simulink model "LIF"  (R2024b)
settings: Solver=ode23t  StartTime=0.0  StopTime=3  MaxStep=1e-05
libraries: fl_lib x15, nesl_utility x5
settings Model: SimulationMode=accelerator  Creator=georg  LastModifiedBy=georg
settings SolverCC: SolverResetMethod=Robust  AutoInsertRateTranBlk=on

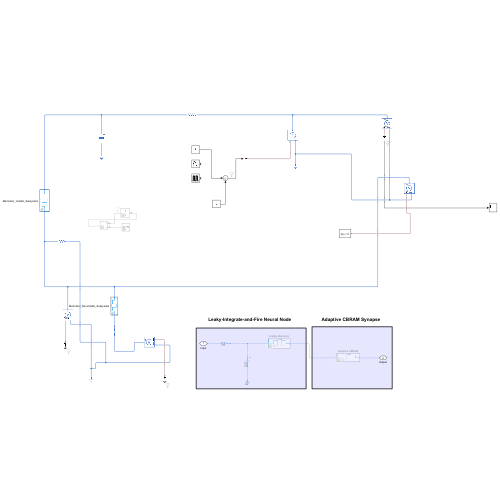
[thumbnail: Simulink's stored preview of the top-level diagram]
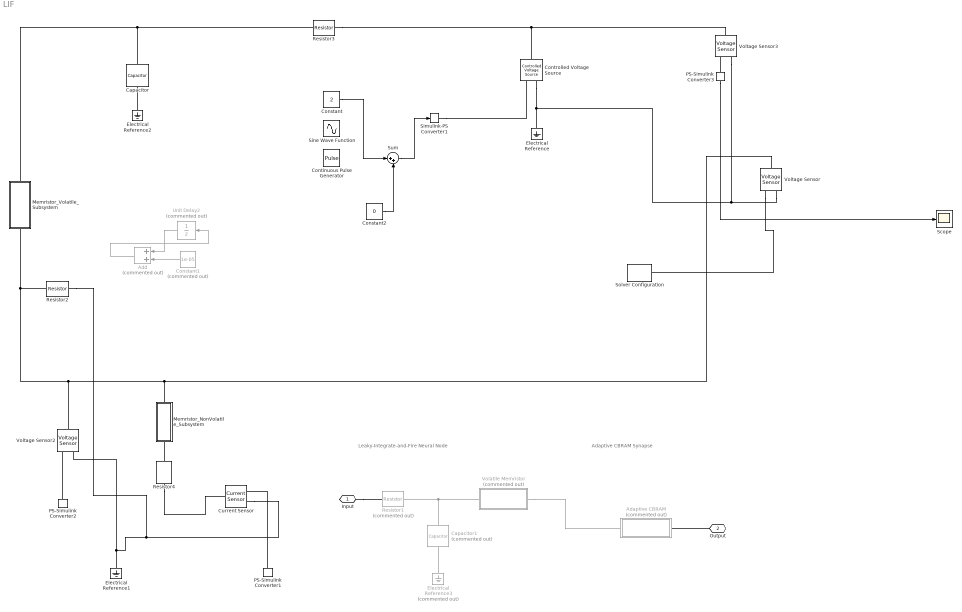
== system LIF ==
  note: Leaky-Integrate-and-Fire Neural Node
  note: Adaptive CBRAM Synapse
  Adaptive CBRAM : Subsystem  Commented=on  ReferencedSubsystem=Memristor_NonVolatile_Subsystem
  Add : Sum  Commented=on
  Capacitor : fl_lib/Electrical/Electrical Elements/Capacitor  c=150 nF  r=1e-6 Ohm  g=0 1/Ohm  i_specify=off  i_priority=None  i=0 A  i_nominal_specify=off  i_nominal_value=1  i_nominal_unit=A  v_specify=off  v_priority=None  v=0 V  v_nominal_specify=off  v_nominal_value=1  v_nominal_unit=V  vc_specify=off  vc_priority=High  vc=0 V  vc_nominal_specify=off  vc_nominal_value=1  vc_nominal_unit=V
  Capacitor1 : fl_lib/Electrical/Electrical Elements/Capacitor  Commented=on  c=150 nF  r=1e-6 Ohm  g=0 1/Ohm  i_specify=off  i_priority=None  i=0 A  i_nominal_specify=off  i_nominal_value=1  i_nominal_unit=A  v_specify=off  v_priority=None  v=0 V  v_nominal_specify=off  v_nominal_value=1  v_nominal_unit=V  vc_specify=off  vc_priority=High  vc=0 V  vc_nominal_specify=off  vc_nominal_value=1  vc_nominal_unit=V
  Constant : Constant  Value=2
  Constant1 : Constant  Commented=on  Value=1e-05
  Constant2 : Constant  Value=0
  Continuous Pulse Generator : DiscretePulseGenerator  PulseType=Time based  Amplitude=2  Period=0.1  PulseWidth=50
  Controlled Voltage Source : fl_lib/Electrical/Electrical Sources/Controlled Voltage Source
  Current Sensor : fl_lib/Electrical/Electrical Sensors/Current Sensor
  Electrical Reference : fl_lib/Electrical/Electrical Elements/Electrical Reference
  Electrical Reference1 : fl_lib/Electrical/Electrical Elements/Electrical Reference
  Electrical Reference2 : fl_lib/Electrical/Electrical Elements/Electrical Reference
  Electrical Reference3 : fl_lib/Electrical/Electrical Elements/Electrical Reference  Commented=on
  Memristor_NonVolatile_Subsystem : Subsystem  ReferencedSubsystem=Memristor_NonVolatile_Subsystem
  Memristor_Volatile_Subsystem : Subsystem  ReferencedSubsystem=Memristor_Volatile_Subsystem
  PS-Simulink Converter1 : nesl_utility/PS-Simulink Converter  PhysicalDomain=network_engine_domain  SubClassName=ps_output  LeftPortType=input  RightPortType=output  PseudoPeriodic=off  Frequencies=[]  VectorFormat=inherit  Unit=inherit  AffineConversion=off
  PS-Simulink Converter2 : nesl_utility/PS-Simulink Converter  PhysicalDomain=network_engine_domain  SubClassName=ps_output  LeftPortType=input  RightPortType=output  PseudoPeriodic=off  Frequencies=[]  VectorFormat=inherit  Unit=inherit  AffineConversion=off
  PS-Simulink Converter3 : nesl_utility/PS-Simulink Converter  PhysicalDomain=network_engine_domain  SubClassName=ps_output  LeftPortType=input  RightPortType=output  PseudoPeriodic=off  Frequencies=[]  VectorFormat=inherit  Unit=inherit  AffineConversion=off
  Resistor1 : fl_lib/Electrical/Electrical Elements/Resistor  Commented=on  R=475 kOhm  i_specify=off  i_priority=None  i=0 A  i_nominal_specify=off  i_nominal_value=1  i_nominal_unit=A  v_specify=off  v_priority=None  v=0 V  v_nominal_specify=off  v_nominal_value=1  v_nominal_unit=V
  Resistor2 : fl_lib/Electrical/Electrical Elements/Resistor  R=0.3 MOhm  i_specify=off  i_priority=None  i=0 A  i_nominal_specify=off  i_nominal_value=1  i_nominal_unit=A  v_specify=off  v_priority=None  v=0 V  v_nominal_specify=off  v_nominal_value=1  v_nominal_unit=V
  Resistor3 : fl_lib/Electrical/Electrical Elements/Resistor  R=475 kOhm  i_specify=off  i_priority=None  i=0 A  i_nominal_specify=off  i_nominal_value=1  i_nominal_unit=A  v_specify=off  v_priority=None  v=0 V  v_nominal_specify=off  v_nominal_value=1  v_nominal_unit=V
  Resistor4 : fl_lib/Electrical/Electrical Elements/Resistor  R=10 kOhm  i_specify=off  i_priority=None  i=0 A  i_nominal_specify=off  i_nominal_value=1  i_nominal_unit=A  v_specify=off  v_priority=None  v=0 V  v_nominal_specify=off  v_nominal_value=1  v_nominal_unit=V
  Scope : Scope
  Simulink-PS Converter1 : nesl_utility/Simulink-PS Converter  PhysicalDomain=network_engine_domain  SubClassName=ps_input  LeftPortType=input  RightPortType=output  PseudoPeriodic=off  Frequencies=[]  NoiseDistribution=none  NoiseParameters=[]  Unit=1  AffineConversion=off  FilteringAndDerivatives=filter  SimscapeFilterOrder=1  InputFilterTimeConstant=0.00001  UdotUserProvided=0
  Sine Wave Function : Sin  Amplitude=2  SampleTime=0
  Solver Configuration : nesl_utility/Solver Configuration  PhysicalDomain=network_engine_domain  SubClassName=solver  LeftPortType=input  RightPortType=generic  Tones=[]  Harmonics=[]  SimulateNoise=off  Profile=off  UseLocalSampling=off  EnableSwitchedLinearOptims=on  FrequencyDomain=off  UseCCode=off  RelTol=0.001  AbsTol=0.001  MinStep=1e-09  ToWorkspace=off  RevertToSquareIcSolve=off  NumHomotopyIterations=100  PhasorMode=off  PhasorModeNumHarmonics=1  ConsistencySolver=NEWTON_XTOL_AFTER_FTOL  IndexReductionMethod=DerivativeReplacement  DoDC=off  ResidualTolerance=1e-09  ConsistencyTolSource=GLOBAL  ConsistencyAbsTol=0.001  ConsistencyRelTol=0.001  ConsistencyTolFactor=0.001  UseLocalSolver=off  LocalSolverChoice=NE_BACKWARD_EULER_ADVANCER  ResolveIndetEquations=on  FunctionEvalNumThread=1  LocalSolverSampleTime=0.001  DoFixedCost=off  MaxNonlinIter=3  MaxModeIter=2  ComputeImpulses=off  ImpulseIterations=2  LinearAlgebra=auto  LinearAlgebraNumThread=0  EquationFormulation=NE_TIME_EF  DelaysMemoryBudget=1024  AutomaticFiltering=on  FilteringTimeConstant=0.001  PartitionStorageMethod=AS_NEEDED  PartitionMemoryBudget=1024  PartitionMethod=ROBUST  MultibodyUseLocalSolver=off  MultibodyLocalSolverChoice=ODE1  MultibodyLocalSolverSampleTime=0.001
  Sum : Sum  Inputs=|++
  Unit Delay2 : UnitDelay  Commented=on  SampleTime=1e-05  HasFrameUpgradeWarning=on
  Volatile Memristor : Subsystem  Commented=on  ReferencedSubsystem=Memristor_Volatile_Subsystem
  Voltage Sensor : fl_lib/Electrical/Electrical Sensors/Voltage Sensor
  Voltage Sensor2 : fl_lib/Electrical/Electrical Sensors/Voltage Sensor
  Voltage Sensor3 : fl_lib/Electrical/Electrical Sensors/Voltage Sensor
  Input : PMIOPort  Side=Left
  Output : PMIOPort  Port=2  Side=Left
  wires:
  PS-Simulink Converter3/1 -> Scope/1
  Constant1/1 -> Add/2
  Unit Delay2/1 -> Add/1
  Add/1 -> Unit Delay2/1
  Constant2/1 -> Sum/2
  Sum/1 -> Simulink-PS Converter1/1
  Constant/1 -> Sum/1
  connections:
  Voltage Sensor/RConn2 -- Voltage Sensor3/RConn2 -- Controlled Voltage Source/RConn2 -- Electrical Reference/LConn1
  Voltage Sensor/RConn1 -- Solver Configuration/RConn1
  Memristor_Volatile_Subsystem/LConn1 -- Capacitor/LConn1 -- Resistor3/LConn1
  Electrical Reference1/LConn1 -- Current Sensor/RConn2 -- Resistor2/RConn1 -- Voltage Sensor2/RConn2
  PS-Simulink Converter2/LConn1 -- Voltage Sensor2/RConn1
  Electrical Reference2/LConn1 -- Capacitor/RConn1
  Controlled Voltage Source/LConn1 -- Resistor3/RConn1 -- Voltage Sensor3/LConn1
  PS-Simulink Converter3/LConn1 -- Voltage Sensor3/RConn1
  Simulink-PS Converter1/RConn1 -- Controlled Voltage Source/RConn1
  PS-Simulink Converter1/LConn1 -- Current Sensor/RConn1
  Voltage Sensor2/LConn1 -- Resistor2/LConn1 -- Memristor_Volatile_Subsystem/RConn1 -- Voltage Sensor/LConn1 -- Memristor_NonVolatile_Subsystem/LConn1
  Resistor4/LConn1 -- Memristor_NonVolatile_Subsystem/RConn1
  Resistor4/RConn1 -- Current Sensor/LConn1
  Volatile Memristor/LConn1 -- Adaptive CBRAM/RConn1
  Volatile Memristor/RConn1 -- Capacitor1/LConn1 -- Resistor1/RConn1
  Electrical Reference3/LConn1 -- Capacitor1/RConn1
  Input/RConn1 -- Resistor1/LConn1
  Output/RConn1 -- Adaptive CBRAM/LConn1
